simulink model "sampleModel153_pp"  (R2021a)
settings: Solver=VariableStepAuto  StartTime=0.0  StopTime=10.0  RelTol=1e-3
undefined symbols (not defined in the file or in its folder): DiscIntNeverNeededParam, magnitude, Newton, Raphson
libraries: simulink x48, pid_lib x19
(part 2 of 3)

== system sampleModel153_pp/cfblk50/cfblk11 ==
  cfblk1 : Inport
  cfblk12 : Inport  Port=2
  cfblk13 : Inport  Port=3
  cfblk10 : Polyval  Coefs=[ +2.081618890e-019, -1.441693666e-014, +4.719686976e-010, -8.536869453e-006, +1.621573104e-001, -8.087801117e+001 ]
  cfblk11 : Constant  Value=[984784884.031660]  SampleTime=1
  cfblk16 : Delay  SampleTime=1
  cfblk3 : DiscreteFir  SampleTime=1
  cfblk4 : pid_lib/PID Controller  Controller=PID  Form=Parallel  TimeDomain=Discrete-time  UseExternalTs=off  SampleTime=1  IntegratorMethod=Forward Euler  FilterMethod=Forward Euler  ControllerParametersSource=internal  P=1  I=1  D=0  UseFilter=on  N=100  TunerSelectOption=Transfer Function Based (PID Tuner App)  InitialConditionSource=internal  InitialConditionForIntegrator=0  InitialConditionForFilter=0  DifferentiatorICPrevScaledInput=0  ExternalReset=none  TrackingMode=off  Kt=1  LimitOutput=off  SatLimitsSource=internal  UpperSaturationLimit=inf  LowerSaturationLimit=-inf  LinearizeAsGain=off  AntiWindupMode=none  Kb=1  POutMin=[]  POutMax=[]  IOutMin=[]  IOutMax=[]  DOutMin=[]  DOutMax=[]  NOutMin=[]  NOutMax=[]  SumOutMin=[]  SumOutMax=[]  SaturationOutMin=[]  SaturationOutMax=[]  PParamMin=[]  PParamMax=[]  IParamMin=[]  IParamMax=[]  DParamMin=[]  DParamMax=[]  NParamMin=[]  NParamMax=[]  KbParamMin=[]  KbParamMax=[]  KtParamMin=[]  KtParamMax=[]  KbOutMin=[]  KbOutMax=[]  KtOutMin=[]  KtOutMax=[]  IntegratorOutMin=[]  IntegratorOutMax=[]  FilterOutMin=[]  FilterOutMax=[]  SumI1OutMin=[]  SumI1OutMax=[]  SumI2OutMin=[]  SumI2OutMax=[]  SumI3OutMin=[]  SumI3OutMax=[]  SumI4OutMin=[]  SumI4OutMax=[]  SumDOutMin=[]  SumDOutMax=[]  DifferentiatorOutMin=[]  DifferentiatorOutMax=[]  FilterDiffOutCoefMin=[]  FilterDiffOutCoefMax=[]  ReciprocalOutMin=[]  ReciprocalOutMax=[]  SumDenOutMin=[]  SumDenOutMax=[]  SumNumOutMin=[]  SumNumOutMax=[]  DivideOutMin=[]  DivideOutMax=[]  UdiffTsProdOutMin=[]  UdiffTsProdOutMax=[]  NTsProdOutMin=[]  NTsProdOutMax=[]  UintegralTsProdOutMin=[]  UintegralTsProdOutMax=[]  UngainTsProdOutMin=[]  UngainTsProdOutMax=[]  IntegratorContinuousStateAttributes=''  IntegratorStateMustResolveToSignalObject=off  IntegratorRTWStateStorageClass=Auto  FilterContinuousStateAttributes=''  FilterStateMustResolveToSignalObject=off  FilterRTWStateStorageClass=Auto  ParallelPVariant=InternalParameters  IdealPVariant=Disabled  IVariant=InternalParameters  DVariant=InternalParameters  IntegratorVariant=Discrete  SatVariant=Disabled  AWVariant=Passthrough  PCopyVariant=Disabled  TRVariant=Disabled  FdbkBlocksVariant=Forward  IdealPFdbkVariant=Disabled  SatFdbkVariant=Disabled  DerivativeFilterVariant=ForwardEulerFilter  NVariant=InternalParameters  NCopyVariant=Disabled  FilterICVariant=InternalICsFilter  IntegratorICVariant=InternalICs  ExternalResetVariant=Disabled  TRSumVariant=Passthrough  SumFdbkVariant=Disabled  SumVariant=Sum_PID  TsampFilterVariant=InternalTs  TsampNgainVariant=Passthrough  TsampIntegralVariant=Passthrough  ExternalSaturationOutDataTypeStr=Inherit: Same as second input
  cfblk5 : Sqrt  Operator=rSqrt  AlgorithmType=Newton-Raphson  SaturateOnIntegerOverflow=on
  cfblk6 : Rounding
  cfblk7 : Trigonometry
  cfblk8 : Assignment  DiagnosticForDimensions=Warning  IndexOptions=Index vector (dialog)  Indices=1  OutputSizes=1
  cfblk9 : MinMax  Function=max  Inputs=3
  cfblk2 : Outport
  cfblk14 : Outport  Port=2
  cfblk15 : Outport  Port=3
  wires:
  cfblk9/1 -> cfblk7/1
  cfblk13/1 -> cfblk2/1, cfblk10/1
  cfblk3/1 -> cfblk6/1
  cfblk6/1 -> cfblk4/1
  cfblk7/1 -> cfblk3/1
  cfblk12/1 -> cfblk8/1
  cfblk8/1 -> cfblk14/1
  cfblk5/1 -> cfblk8/2, cfblk9/3
  cfblk11/1 -> cfblk5/1
  cfblk1/1 -> cfblk9/1
  cfblk10/1 -> cfblk15/1
  cfblk4/1 -> cfblk16/1
  cfblk16/1 -> cfblk9/2

== system sampleModel153_pp/cfblk50/cfblk12 ==
  cfblk1 : Inport
  cfblk6 : Inport  Port=2
  cfblk3 : ComplexToMagnitudeAngle
  cfblk4 : Sqrt  SaturateOnIntegerOverflow=on
  cfblk5 : Constant  Value=[784222479.091064]  SampleTime=1
  cfblk2 : Outport
  cfblk7 : Outport  Port=2
  wires:
  cfblk1/1 -> cfblk4/1
  cfblk6/1 -> cfblk3/1
  cfblk3/1 -> cfblk7/1
  cfblk3/2 -> cfblk2/1

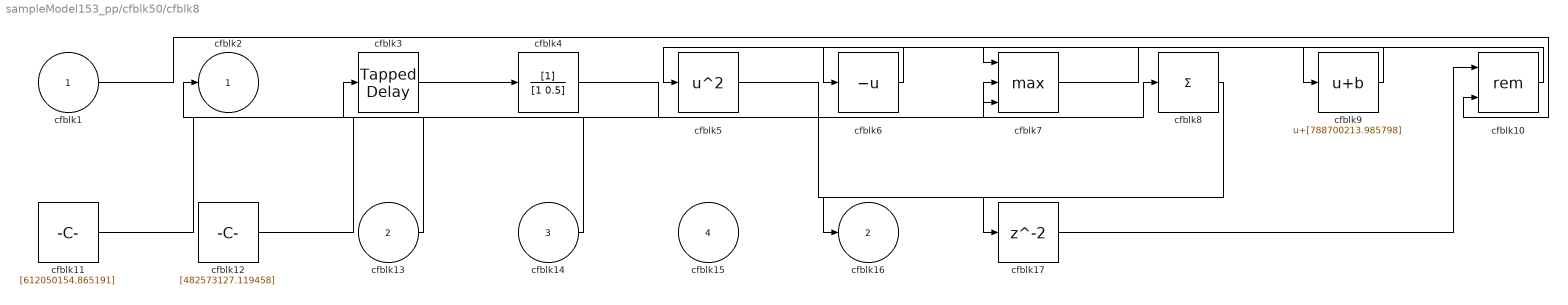
== system sampleModel153_pp/cfblk50/cfblk8 ==
  cfblk1 : Inport
  cfblk13 : Inport  Port=2
  cfblk14 : Inport  Port=3
  cfblk15 : Inport  Port=4
  cfblk10 : Math  Operator=rem  SaturateOnIntegerOverflow=on
  cfblk11 : Constant  Value=[612050154.865191]  SampleTime=1
  cfblk12 : Constant  Value=[482573127.119458]  SampleTime=1
  cfblk17 : Delay  SampleTime=1
  cfblk3 : simulink/Discrete/Tapped Delay  vinit=0.0  samptime=-1  NumDelays=1  DelayOrder=Oldest  includeCurrent=off
  cfblk4 : DiscreteFilter  SampleTime=1
  cfblk5 : Math  Operator=square  SaturateOnIntegerOverflow=on
  cfblk6 : UnaryMinus
  cfblk7 : MinMax  Function=max  Inputs=3
  cfblk8 : Sum  Inputs=+
  cfblk9 : Bias  Bias=[788700213.985798]
  cfblk2 : Outport
  cfblk16 : Outport  Port=2
  wires:
  cfblk11/1 -> cfblk8/1
  cfblk6/1 -> cfblk5/1
  cfblk3/1 -> cfblk4/1
  cfblk10/1 -> cfblk7/1
  cfblk12/1 -> cfblk7/2
  cfblk8/1 -> cfblk16/1
  cfblk14/1 -> cfblk3/1
  cfblk4/1 -> cfblk7/3
  cfblk7/1 -> cfblk9/1
  cfblk9/1 -> cfblk6/1
  cfblk13/1 -> cfblk2/1
  cfblk1/1 -> cfblk10/2
  cfblk5/1 -> cfblk17/1
  cfblk17/1 -> cfblk10/1

== system sampleModel153_pp/cfblk50/cfblk9 ==
  cfblk1 : Inport
  cfblk3 : DiscreteIntegrator  ICPrevOutput=DiscIntNeverNeededParam  ICPrevScaledInput=DiscIntNeverNeededParam
  cfblk4 : Delay  ShowEnablePort=on  SampleTime=1
      settings: InputPortMap=u0,e6
  cfblk5 : DiscreteFir  SampleTime=1
  cfblk6 : DiscreteIntegrator  ICPrevOutput=DiscIntNeverNeededParam  ICPrevScaledInput=DiscIntNeverNeededParam
  cfblk7 : PermuteDimensions
  cfblk8 : Delay  SampleTime=1
  cfblk2 : Outport
  wires:
  cfblk5/1 -> cfblk2/1
  cfblk4/1 -> cfblk3/1
  cfblk7/1 -> cfblk4/1
  cfblk1/1 -> cfblk7/1
  cfblk6/1 -> cfblk5/1, cfblk8/1
  cfblk3/1 -> cfblk6/1
  cfblk8/1 -> cfblk4/2

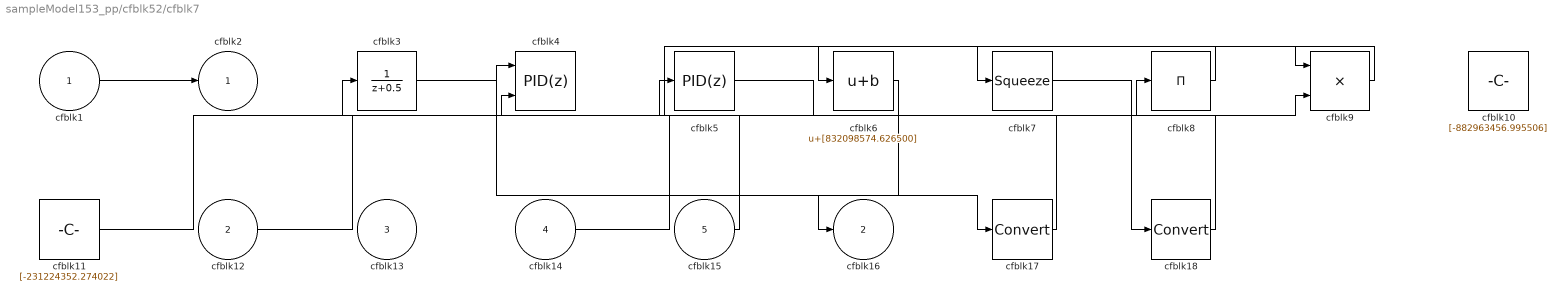
== system sampleModel153_pp/cfblk52/cfblk7 ==
  cfblk1 : Inport
  cfblk12 : Inport  Port=2
  cfblk13 : Inport  Port=3
  cfblk14 : Inport  Port=4
  cfblk15 : Inport  Port=5
  cfblk10 : Constant  Value=[-882963456.995506]  SampleTime=1
  cfblk11 : Constant  Value=[-231224352.274022]  SampleTime=1
  cfblk17 : DataTypeConversion
  cfblk18 : DataTypeConversion
  cfblk3 : DiscreteTransferFcn  SampleTime=1
  cfblk4 : pid_lib/PID Controller (2DOF)  Controller=PID  Form=Parallel  TimeDomain=Discrete-time  UseExternalTs=off  SampleTime=1  IntegratorMethod=Forward Euler  FilterMethod=Forward Euler  ControllerParametersSource=internal  P=1  I=1  D=0  UseFilter=on  N=100  b=1  c=1  TunerSelectOption=Transfer Function Based (PID Tuner App)  InitialConditionSource=internal  InitialConditionForIntegrator=0  InitialConditionForFilter=0  DifferentiatorICPrevScaledInput=0  ExternalReset=none  TrackingMode=off  Kt=1  LimitOutput=off  SatLimitsSource=internal  UpperSaturationLimit=inf  LowerSaturationLimit=-inf  LinearizeAsGain=off  AntiWindupMode=none  Kb=1  POutMin=[]  POutMax=[]  IOutMin=[]  IOutMax=[]  DOutMin=[]  DOutMax=[]  NOutMin=[]  NOutMax=[]  bOutMin=[]  bOutMax=[]  cOutMin=[]  cOutMax=[]  SumOutMin=[]  SumOutMax=[]  SaturationOutMin=[]  SaturationOutMax=[]  PParamMin=[]  PParamMax=[]  IParamMin=[]  IParamMax=[]  DParamMin=[]  DParamMax=[]  NParamMin=[]  NParamMax=[]  bParamMin=[]  bParamMax=[]  cParamMin=[]  cParamMax=[]  KbParamMin=[]  KbParamMax=[]  KtParamMin=[]  KtParamMax=[]  KbOutMin=[]  KbOutMax=[]  KtOutMin=[]  KtOutMax=[]  IntegratorOutMin=[]  IntegratorOutMax=[]  FilterOutMin=[]  FilterOutMax=[]  SumI1OutMin=[]  SumI1OutMax=[]  SumI2OutMin=[]  SumI2OutMax=[]  SumI3OutMin=[]  SumI3OutMax=[]  SumI4OutMin=[]  SumI4OutMax=[]  SumDOutMin=[]  SumDOutMax=[]  Sum1OutMin=[]  Sum1OutMax=[]  Sum2OutMin=[]  Sum2OutMax=[]  Sum3OutMin=[]  Sum3OutMax=[]  DifferentiatorOutMin=[]  DifferentiatorOutMax=[]  FilterDiffOutCoefMin=[]  FilterDiffOutCoefMax=[]  ReciprocalOutMin=[]  ReciprocalOutMax=[]  SumDenOutMin=[]  SumDenOutMax=[]  SumNumOutMin=[]  SumNumOutMax=[]  DivideOutMin=[]  DivideOutMax=[]  UdiffTsProdOutMin=[]  UdiffTsProdOutMax=[]  NTsProdOutMin=[]  NTsProdOutMax=[]  UintegralTsProdOutMin=[]  UintegralTsProdOutMax=[]  UngainTsProdOutMin=[]  UngainTsProdOutMax=[]  IntegratorContinuousStateAttributes=''  IntegratorStateMustResolveToSignalObject=off  IntegratorRTWStateStorageClass=Auto  FilterContinuousStateAttributes=''  FilterStateMustResolveToSignalObject=off  FilterRTWStateStorageClass=Auto  ParallelPVariant=InternalParameters  IdealPVariant=Disabled  IVariant=InternalParameters  DVariant=InternalParameters  bVariant=InternalParameters  cVariant=InternalParameters  IntegratorVariant=Discrete  SatVariant=Disabled  AWVariant=Passthrough  PCopyVariant=Disabled  TRVariant=Disabled  FdbkBlocksVariant=Forward  IdealPFdbkVariant=Disabled  SatFdbkVariant=Disabled  DerivativeFilterVariant=ForwardEulerFilter  NVariant=InternalParameters  NCopyVariant=Disabled  FilterICVariant=InternalICsFilter  IntegratorICVariant=InternalICs  ExternalResetVariant=Disabled  TRSumVariant=Passthrough  SumFdbkVariant=Disabled  SumVariant=Sum_PID  TsampFilterVariant=InternalTs  TsampNgainVariant=Passthrough  TsampIntegralVariant=Passthrough  ExternalSaturationOutDataTypeStr=Inherit: Same as second input
      settings: SourceProductBaseCode=SL
  cfblk5 : pid_lib/PID Controller  Controller=PID  Form=Parallel  TimeDomain=Discrete-time  UseExternalTs=off  SampleTime=1  IntegratorMethod=Forward Euler  FilterMethod=Forward Euler  ControllerParametersSource=internal  P=1  I=1  D=0  UseFilter=on  N=100  TunerSelectOption=Transfer Function Based (PID Tuner App)  InitialConditionSource=internal  InitialConditionForIntegrator=0  InitialConditionForFilter=0  DifferentiatorICPrevScaledInput=0  ExternalReset=none  TrackingMode=off  Kt=1  LimitOutput=off  SatLimitsSource=internal  UpperSaturationLimit=inf  LowerSaturationLimit=-inf  LinearizeAsGain=off  AntiWindupMode=none  Kb=1  POutMin=[]  POutMax=[]  IOutMin=[]  IOutMax=[]  DOutMin=[]  DOutMax=[]  NOutMin=[]  NOutMax=[]  SumOutMin=[]  SumOutMax=[]  SaturationOutMin=[]  SaturationOutMax=[]  PParamMin=[]  PParamMax=[]  IParamMin=[]  IParamMax=[]  DParamMin=[]  DParamMax=[]  NParamMin=[]  NParamMax=[]  KbParamMin=[]  KbParamMax=[]  KtParamMin=[]  KtParamMax=[]  KbOutMin=[]  KbOutMax=[]  KtOutMin=[]  KtOutMax=[]  IntegratorOutMin=[]  IntegratorOutMax=[]  FilterOutMin=[]  FilterOutMax=[]  SumI1OutMin=[]  SumI1OutMax=[]  SumI2OutMin=[]  SumI2OutMax=[]  SumI3OutMin=[]  SumI3OutMax=[]  SumI4OutMin=[]  SumI4OutMax=[]  SumDOutMin=[]  SumDOutMax=[]  DifferentiatorOutMin=[]  DifferentiatorOutMax=[]  FilterDiffOutCoefMin=[]  FilterDiffOutCoefMax=[]  ReciprocalOutMin=[]  ReciprocalOutMax=[]  SumDenOutMin=[]  SumDenOutMax=[]  SumNumOutMin=[]  SumNumOutMax=[]  DivideOutMin=[]  DivideOutMax=[]  UdiffTsProdOutMin=[]  UdiffTsProdOutMax=[]  NTsProdOutMin=[]  NTsProdOutMax=[]  UintegralTsProdOutMin=[]  UintegralTsProdOutMax=[]  UngainTsProdOutMin=[]  UngainTsProdOutMax=[]  IntegratorContinuousStateAttributes=''  IntegratorStateMustResolveToSignalObject=off  IntegratorRTWStateStorageClass=Auto  FilterContinuousStateAttributes=''  FilterStateMustResolveToSignalObject=off  FilterRTWStateStorageClass=Auto  ParallelPVariant=InternalParameters  IdealPVariant=Disabled  IVariant=InternalParameters  DVariant=InternalParameters  IntegratorVariant=Discrete  SatVariant=Disabled  AWVariant=Passthrough  PCopyVariant=Disabled  TRVariant=Disabled  FdbkBlocksVariant=Forward  IdealPFdbkVariant=Disabled  SatFdbkVariant=Disabled  DerivativeFilterVariant=ForwardEulerFilter  NVariant=InternalParameters  NCopyVariant=Disabled  FilterICVariant=InternalICsFilter  IntegratorICVariant=InternalICs  ExternalResetVariant=Disabled  TRSumVariant=Passthrough  SumFdbkVariant=Disabled  SumVariant=Sum_PID  TsampFilterVariant=InternalTs  TsampNgainVariant=Passthrough  TsampIntegralVariant=Passthrough  ExternalSaturationOutDataTypeStr=Inherit: Same as second input
  cfblk6 : Bias  Bias=[832098574.626500]
  cfblk7 : Squeeze
  cfblk8 : Product  Inputs=*
  cfblk9 : Product  Inputs=**
  cfblk2 : Outport
  cfblk16 : Outport  Port=2
  wires:
  cfblk14/1 -> cfblk8/1
  cfblk12/1 -> cfblk9/1
  cfblk6/1 -> cfblk16/1
  cfblk15/1 -> cfblk5/1
  cfblk1/1 -> cfblk2/1
  cfblk9/1 -> cfblk6/1
  cfblk11/1 -> cfblk4/2
  cfblk8/1 -> cfblk7/1
  cfblk5/1 -> cfblk9/2
  cfblk3/1 -> cfblk17/1
  cfblk17/1 -> cfblk4/1
  cfblk7/1 -> cfblk18/1
  cfblk18/1 -> cfblk3/1

== system sampleModel153_pp/cfblk53/cfblk11 ==
  cfblk1 : Inport
  cfblk9 : Inport  Port=2
  cfblk10 : Inport  Port=3
  cfblk11 : Inport  Port=4
  cfblk3 : DiscreteZeroPole  Poles=[0 0.5]  Gain=1
  cfblk4 : pid_lib/PID Controller  Controller=PID  Form=Parallel  TimeDomain=Discrete-time  UseExternalTs=off  SampleTime=1  IntegratorMethod=Forward Euler  FilterMethod=Forward Euler  ControllerParametersSource=internal  P=1  I=1  D=0  UseFilter=on  N=100  TunerSelectOption=Transfer Function Based (PID Tuner App)  InitialConditionSource=internal  InitialConditionForIntegrator=0  InitialConditionForFilter=0  DifferentiatorICPrevScaledInput=0  ExternalReset=none  TrackingMode=off  Kt=1  LimitOutput=off  SatLimitsSource=internal  UpperSaturationLimit=inf  LowerSaturationLimit=-inf  LinearizeAsGain=off  AntiWindupMode=none  Kb=1  POutMin=[]  POutMax=[]  IOutMin=[]  IOutMax=[]  DOutMin=[]  DOutMax=[]  NOutMin=[]  NOutMax=[]  SumOutMin=[]  SumOutMax=[]  SaturationOutMin=[]  SaturationOutMax=[]  PParamMin=[]  PParamMax=[]  IParamMin=[]  IParamMax=[]  DParamMin=[]  DParamMax=[]  NParamMin=[]  NParamMax=[]  KbParamMin=[]  KbParamMax=[]  KtParamMin=[]  KtParamMax=[]  KbOutMin=[]  KbOutMax=[]  KtOutMin=[]  KtOutMax=[]  IntegratorOutMin=[]  IntegratorOutMax=[]  FilterOutMin=[]  FilterOutMax=[]  SumI1OutMin=[]  SumI1OutMax=[]  SumI2OutMin=[]  SumI2OutMax=[]  SumI3OutMin=[]  SumI3OutMax=[]  SumI4OutMin=[]  SumI4OutMax=[]  SumDOutMin=[]  SumDOutMax=[]  DifferentiatorOutMin=[]  DifferentiatorOutMax=[]  FilterDiffOutCoefMin=[]  FilterDiffOutCoefMax=[]  ReciprocalOutMin=[]  ReciprocalOutMax=[]  SumDenOutMin=[]  SumDenOutMax=[]  SumNumOutMin=[]  SumNumOutMax=[]  DivideOutMin=[]  DivideOutMax=[]  UdiffTsProdOutMin=[]  UdiffTsProdOutMax=[]  NTsProdOutMin=[]  NTsProdOutMax=[]  UintegralTsProdOutMin=[]  UintegralTsProdOutMax=[]  UngainTsProdOutMin=[]  UngainTsProdOutMax=[]  IntegratorContinuousStateAttributes=''  IntegratorStateMustResolveToSignalObject=off  IntegratorRTWStateStorageClass=Auto  FilterContinuousStateAttributes=''  FilterStateMustResolveToSignalObject=off  FilterRTWStateStorageClass=Auto  ParallelPVariant=InternalParameters  IdealPVariant=Disabled  IVariant=InternalParameters  DVariant=InternalParameters  IntegratorVariant=Discrete  SatVariant=Disabled  AWVariant=Passthrough  PCopyVariant=Disabled  TRVariant=Disabled  FdbkBlocksVariant=Forward  IdealPFdbkVariant=Disabled  SatFdbkVariant=Disabled  DerivativeFilterVariant=ForwardEulerFilter  NVariant=InternalParameters  NCopyVariant=Disabled  FilterICVariant=InternalICsFilter  IntegratorICVariant=InternalICs  ExternalResetVariant=Disabled  TRSumVariant=Passthrough  SumFdbkVariant=Disabled  SumVariant=Sum_PID  TsampFilterVariant=InternalTs  TsampNgainVariant=Passthrough  TsampIntegralVariant=Passthrough  ExternalSaturationOutDataTypeStr=Inherit: Same as second input
  cfblk5 : Abs
  cfblk6 : Sum  Inputs=|++
  cfblk7 : Signum
  cfblk8 : Abs
  cfblk2 : Outport
  cfblk12 : Outport  Port=2
  wires:
  cfblk9/1 -> cfblk8/1
  cfblk5/1 -> cfblk12/1
  cfblk8/1 -> cfblk4/1
  cfblk1/1 -> cfblk3/1
  cfblk3/1 -> cfblk6/1
  cfblk11/1 -> cfblk7/1
  cfblk4/1 -> cfblk2/1
  cfblk6/1 -> cfblk5/1
  cfblk10/1 -> cfblk6/2

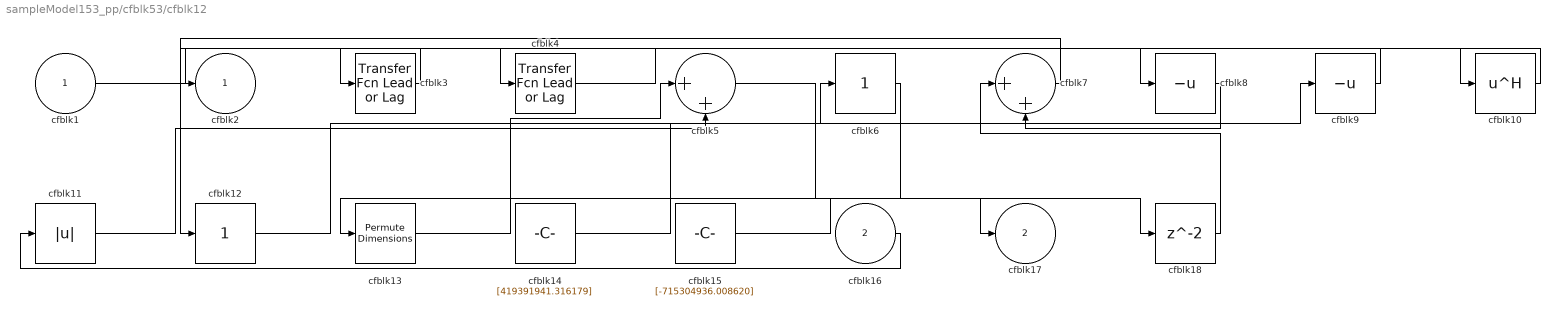
== system sampleModel153_pp/cfblk53/cfblk12 ==
  cfblk1 : Inport
  cfblk16 : Inport  Port=2
  cfblk10 : Math  Operator=hermitian  SaturateOnIntegerOverflow=on
  cfblk11 : Abs
  cfblk12 : simulink/Math Operations/Slider Gain  gain=1  low=0  high=2
  cfblk13 : PermuteDimensions
  cfblk14 : Constant  Value=[419391941.316179]  SampleTime=1
  cfblk15 : Constant  Value=[-715304936.008620]  SampleTime=1
  cfblk18 : Delay  SampleTime=1
  cfblk3 : simulink/Discrete/Transfer Fcn Lead or Lag  PoleZ=0.95  ZeroZ=0.75  ICPrevOutput=0.0  ICPrevInput=0.0  DoSatur=off
      settings: SourceProductBaseCode=SL
  cfblk4 : simulink/Discrete/Transfer Fcn Lead or Lag  PoleZ=0.95  ZeroZ=0.75  ICPrevOutput=0.0  ICPrevInput=0.0  DoSatur=off
      settings: SourceProductBaseCode=SL
  cfblk5 : Sum  Inputs=|++
  cfblk6 : simulink/Math Operations/Slider Gain  gain=1  low=0  high=2
  cfblk7 : Sum  Inputs=|++
  cfblk8 : UnaryMinus
  cfblk9 : UnaryMinus
  cfblk2 : Outport
  cfblk17 : Outport  Port=2
  wires:
  cfblk6/1 -> cfblk13/1
  cfblk16/1 -> cfblk11/1
  cfblk7/1 -> cfblk12/1
  cfblk1/1 -> cfblk4/1
  cfblk12/1 -> cfblk6/1
  cfblk14/1 -> cfblk9/1
  cfblk13/1 -> cfblk5/1
  cfblk11/1 -> cfblk5/2
  cfblk10/1 -> cfblk8/1
  cfblk9/1 -> cfblk3/1
  cfblk3/1 -> cfblk2/1
  cfblk8/1 -> cfblk7/2
  cfblk4/1 -> cfblk10/1
  cfblk15/1 -> cfblk17/1
  cfblk5/1 -> cfblk18/1
  cfblk18/1 -> cfblk7/1

== system sampleModel153_pp/cfblk53/cfblk13 ==
  cfblk1 : Inport
  cfblk12 : Inport  Port=2
  cfblk10 : Sum  Inputs=|++
  cfblk11 : Sum  Inputs=-+
  cfblk14 : Delay  SampleTime=1
  cfblk15 : Delay  SampleTime=1
  cfblk3 : DiscreteFilter  SampleTime=1
  cfblk4 : Delay  DelayLengthSource=Input port  SampleTime=1
      settings: InputPortMap=u0,p1
  cfblk5 : simulink/Math Operations/Slider Gain  gain=1  low=0  high=2
  cfblk6 : Signum
  cfblk7 : simulink/Math Operations/Slider Gain  gain=1  low=0  high=2
  cfblk8 : MinMax  Function=max
  cfblk9 : Gain  Gain=[-990877030.990551]
  cfblk2 : Outport
  cfblk13 : Outport  Port=2
  wires:
  cfblk12/1 -> cfblk13/1
  cfblk3/1 -> cfblk7/1
  cfblk4/1 -> cfblk11/1
  cfblk5/1 -> cfblk4/1
  cfblk9/1 -> cfblk3/1, cfblk8/1
  cfblk1/1 -> cfblk5/1, cfblk11/2
  cfblk11/1 -> cfblk10/1
  cfblk6/1 -> cfblk2/1, cfblk14/1
  cfblk10/1 -> cfblk9/1
  cfblk7/1 -> cfblk6/1
  cfblk14/1 -> cfblk10/2
  cfblk8/1 -> cfblk15/1
  cfblk15/1 -> cfblk4/2

== system sampleModel153_pp/cfblk53/cfblk14 ==
  cfblk1 : Inport
  cfblk6 : Inport  Port=2
  cfblk7 : Inport  Port=3
  cfblk3 : Rounding
  cfblk4 : PermuteDimensions
  cfblk5 : Abs
  cfblk2 : Outport
  cfblk8 : Outport  Port=2
  cfblk9 : Outport  Port=3
  cfblk10 : Outport  Port=4
  wires:
  cfblk1/1 -> cfblk5/1
  cfblk6/1 -> cfblk3/1, cfblk8/1
  cfblk4/1 -> cfblk2/1
  cfblk7/1 -> cfblk4/1
  cfblk5/1 -> cfblk9/1
  cfblk3/1 -> cfblk10/1

== system sampleModel153_pp/cfblk54/cfblk10 ==
  cfblk1 : Inport
  cfblk6 : Inport  Port=2
  cfblk7 : Inport  Port=3
  cfblk3 : simulink/Math Operations/MinMax Running Resettable  Function=min  vinit=0.0
  cfblk4 : Math  Operator=10^u  SaturateOnIntegerOverflow=on
  cfblk5 : Constant  Value=[175787180.328287]  SampleTime=1
  cfblk2 : Outport
  wires:
  cfblk5/1 -> cfblk4/1
  cfblk1/1 -> cfblk2/1
  cfblk4/1 -> cfblk3/1
  cfblk7/1 -> cfblk3/2

== system sampleModel153_pp/cfblk54/cfblk9 ==
  cfblk1 : Inport
  cfblk7 : Inport  Port=2
  cfblk8 : Inport  Port=3
  cfblk9 : Inport  Port=4
  cfblk3 : MinMax
  cfblk4 : Sum  Inputs=+-
  cfblk5 : Constant  Value=[696083638.392896]  SampleTime=1
  cfblk6 : Constant  Value=[-943413520.020544]  SampleTime=1
  cfblk2 : Outport
  wires:
  cfblk4/1 -> cfblk3/1
  cfblk3/1 -> cfblk2/1
  cfblk1/1 -> cfblk4/1
  cfblk5/1 -> cfblk4/2

== system sampleModel153_pp/cfblk55/cfblk10 ==
  cfblk1 : Inport
  cfblk8 : Inport  Port=2
  cfblk3 : Sum  Inputs=+-
  cfblk4 : Sum  Inputs=+
  cfblk5 : MinMax  Function=max
  cfblk6 : Constant  Value=[519421794.730355]  SampleTime=1
  cfblk7 : Constant  Value=[668195430.515494]  SampleTime=1
  cfblk2 : Outport
  wires:
  cfblk7/1 -> cfblk2/1
  cfblk4/1 -> cfblk5/1
  cfblk6/1 -> cfblk4/1
  cfblk8/1 -> cfblk3/1
  cfblk1/1 -> cfblk3/2

== system sampleModel153_pp/cfblk55/cfblk7 ==
  cfblk1 : Inport
  cfblk9 : Inport  Port=2
  cfblk10 : Inport  Port=3
  cfblk11 : Inport  Port=4
  cfblk12 : Inport  Port=5
  cfblk3 : simulink/Discrete/Difference  ICPrevInput=0.0  OutMin=[]  OutMax=[]  OutDataTypeStr=Inherit: Inherit via back propagation  OutDataType=fixdt(1, 16)  OutScaling=2^-10  DoSatur=off
  cfblk4 : Sum  Inputs=+
  cfblk5 : Sum  Inputs=--
  cfblk6 : ComplexToMagnitudeAngle
  cfblk7 : Rounding
  cfblk8 : Reshape
  cfblk2 : Outport
  cfblk13 : Outport  Port=2
  wires:
  cfblk9/1 -> cfblk7/1
  cfblk4/1 -> cfblk6/1
  cfblk8/1 -> cfblk5/1
  cfblk12/1 -> cfblk4/1
  cfblk11/1 -> cfblk3/1
  cfblk1/1 -> cfblk13/1
  cfblk3/1 -> cfblk5/2
  cfblk6/1 -> cfblk8/1
  cfblk10/1 -> cfblk2/1

== system sampleModel153_pp/cfblk55/cfblk8 ==
  cfblk1 : Inport
  cfblk9 : Inport  Port=2
  cfblk12 : Delay  SampleTime=1
  cfblk3 : Rounding
  cfblk4 : Gain  Gain=[218095897.215768]
  cfblk5 : Rounding
  cfblk6 : ComplexToMagnitudeAngle
  cfblk7 : Product  Inputs=*
  cfblk8 : Sum  Inputs=|++
  cfblk2 : Outport
  cfblk10 : Outport  Port=2
  cfblk11 : Outport  Port=3
  wires:
  cfblk8/1 -> cfblk7/1
  cfblk1/1 -> cfblk4/1
  cfblk6/1 -> cfblk3/1
  cfblk6/2 -> cfblk10/1
  cfblk3/1 -> cfblk8/1
  cfblk7/1 -> cfblk5/1, cfblk2/1
  cfblk4/1 -> cfblk6/1
  cfblk9/1 -> cfblk11/1
  cfblk5/1 -> cfblk12/1
  cfblk12/1 -> cfblk8/2

== system sampleModel153_pp/cfblk55/cfblk9 ==
  cfblk1 : Inport
  cfblk9 : Inport  Port=2
  cfblk10 : Inport  Port=3
  cfblk11 : Inport  Port=4
  cfblk12 : Inport  Port=5
  cfblk13 : Inport  Port=6
  cfblk3 : pid_lib/PID Controller  Controller=PID  Form=Parallel  TimeDomain=Discrete-time  UseExternalTs=off  SampleTime=1  IntegratorMethod=Forward Euler  FilterMethod=Forward Euler  ControllerParametersSource=internal  P=1  I=1  D=0  UseFilter=on  N=100  TunerSelectOption=Transfer Function Based (PID Tuner App)  InitialConditionSource=internal  InitialConditionForIntegrator=0  InitialConditionForFilter=0  DifferentiatorICPrevScaledInput=0  ExternalReset=none  TrackingMode=off  Kt=1  LimitOutput=off  SatLimitsSource=internal  UpperSaturationLimit=inf  LowerSaturationLimit=-inf  LinearizeAsGain=off  AntiWindupMode=none  Kb=1  POutMin=[]  POutMax=[]  IOutMin=[]  IOutMax=[]  DOutMin=[]  DOutMax=[]  NOutMin=[]  NOutMax=[]  SumOutMin=[]  SumOutMax=[]  SaturationOutMin=[]  SaturationOutMax=[]  PParamMin=[]  PParamMax=[]  IParamMin=[]  IParamMax=[]  DParamMin=[]  DParamMax=[]  NParamMin=[]  NParamMax=[]  KbParamMin=[]  KbParamMax=[]  KtParamMin=[]  KtParamMax=[]  KbOutMin=[]  KbOutMax=[]  KtOutMin=[]  KtOutMax=[]  IntegratorOutMin=[]  IntegratorOutMax=[]  FilterOutMin=[]  FilterOutMax=[]  SumI1OutMin=[]  SumI1OutMax=[]  SumI2OutMin=[]  SumI2OutMax=[]  SumI3OutMin=[]  SumI3OutMax=[]  SumI4OutMin=[]  SumI4OutMax=[]  SumDOutMin=[]  SumDOutMax=[]  DifferentiatorOutMin=[]  DifferentiatorOutMax=[]  FilterDiffOutCoefMin=[]  FilterDiffOutCoefMax=[]  ReciprocalOutMin=[]  ReciprocalOutMax=[]  SumDenOutMin=[]  SumDenOutMax=[]  SumNumOutMin=[]  SumNumOutMax=[]  DivideOutMin=[]  DivideOutMax=[]  UdiffTsProdOutMin=[]  UdiffTsProdOutMax=[]  NTsProdOutMin=[]  NTsProdOutMax=[]  UintegralTsProdOutMin=[]  UintegralTsProdOutMax=[]  UngainTsProdOutMin=[]  UngainTsProdOutMax=[]  IntegratorContinuousStateAttributes=''  IntegratorStateMustResolveToSignalObject=off  IntegratorRTWStateStorageClass=Auto  FilterContinuousStateAttributes=''  FilterStateMustResolveToSignalObject=off  FilterRTWStateStorageClass=Auto  ParallelPVariant=InternalParameters  IdealPVariant=Disabled  IVariant=InternalParameters  DVariant=InternalParameters  IntegratorVariant=Discrete  SatVariant=Disabled  AWVariant=Passthrough  PCopyVariant=Disabled  TRVariant=Disabled  FdbkBlocksVariant=Forward  IdealPFdbkVariant=Disabled  SatFdbkVariant=Disabled  DerivativeFilterVariant=ForwardEulerFilter  NVariant=InternalParameters  NCopyVariant=Disabled  FilterICVariant=InternalICsFilter  IntegratorICVariant=InternalICs  ExternalResetVariant=Disabled  TRSumVariant=Passthrough  SumFdbkVariant=Disabled  SumVariant=Sum_PID  TsampFilterVariant=InternalTs  TsampNgainVariant=Passthrough  TsampIntegralVariant=Passthrough  ExternalSaturationOutDataTypeStr=Inherit: Same as second input
  cfblk4 : Sqrt  SaturateOnIntegerOverflow=on
  cfblk5 : Sin  TimeSource=Use external signal  SampleTime=0
  cfblk6 : Constant  Value=[-874027630.229869]  SampleTime=1
  cfblk7 : Constant  Value=[-999264160.149922]  SampleTime=1
  cfblk8 : Constant  Value=[958342791.090826]  SampleTime=1
  cfblk2 : Outport
  cfblk14 : Outport  Port=2
  wires:
  cfblk7/1 -> cfblk4/1
  cfblk1/1 -> cfblk5/1
  cfblk12/1 -> cfblk2/1
  cfblk3/1 -> cfblk14/1
  cfblk5/1 -> cfblk3/1

== system sampleModel153_pp/cfblk56/cfblk7 ==
  cfblk1 : Inport
  cfblk10 : Inport  Port=2
  cfblk11 : Inport  Port=3
  cfblk12 : Inport  Port=4
  cfblk13 : Inport  Port=5
  cfblk3 : UnitDelay  HasFrameUpgradeWarning=on
  cfblk4 : Delay  ShowEnablePort=on  SampleTime=1
      settings: InputPortMap=u0,e6
  cfblk5 : simulink/Discrete/Transfer Fcn Real Zero  ZeroZ=0.75  ICPrevInput=0.0  DoSatur=off
      settings: SourceProductBaseCode=SL
  cfblk6 : PermuteDimensions
  cfblk7 : Assignment  DiagnosticForDimensions=Warning  IndexOptions=Index vector (dialog)  Indices=1  OutputSizes=1
  cfblk8 : Constant  Value=[-59489138.603640]  SampleTime=1
  cfblk9 : Constant  Value=[610527409.433895]  SampleTime=1
  cfblk2 : Outport
  wires:
  cfblk3/1 -> cfblk4/1
  cfblk9/1 -> cfblk4/2
  cfblk10/1 -> cfblk5/1
  cfblk12/1 -> cfblk2/1
  cfblk11/1 -> cfblk6/1
  cfblk13/1 -> cfblk7/1
  cfblk4/1 -> cfblk7/2
  cfblk6/1 -> cfblk3/1

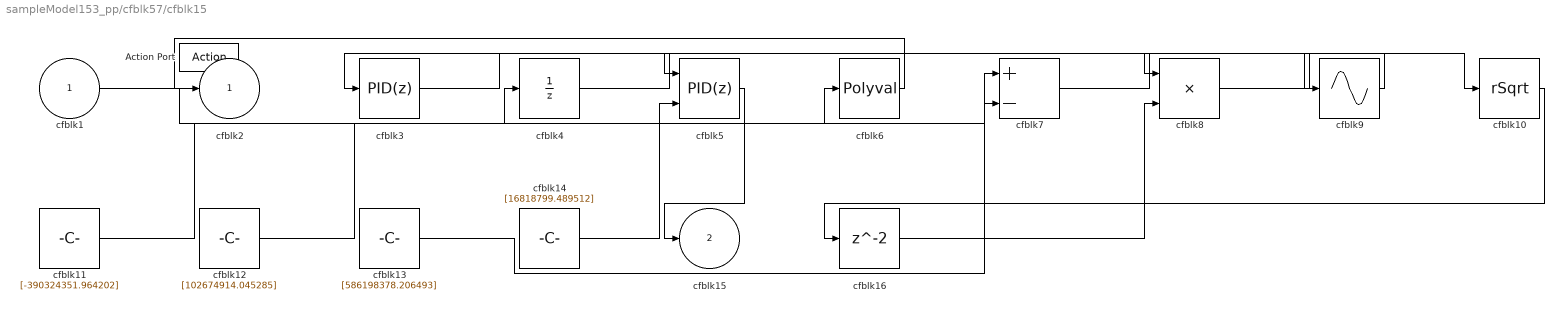
== system sampleModel153_pp/cfblk57/cfblk15 ==
  cfblk1 : Inport
  Action Port : ActionPort  ActionPortLabel=if(u1 >= 0)
  cfblk10 : Sqrt  Operator=rSqrt  AlgorithmType=Newton-Raphson  SaturateOnIntegerOverflow=on
  cfblk11 : Constant  Value=[-390324351.964202]  SampleTime=1
  cfblk12 : Constant  Value=[102674914.045285]  SampleTime=1
  cfblk13 : Constant  Value=[586198378.206493]  SampleTime=1
  cfblk14 : Constant  Value=[16818799.489512]  SampleTime=1
  cfblk16 : Delay
  cfblk3 : pid_lib/PID Controller  Controller=PID  Form=Parallel  TimeDomain=Discrete-time  UseExternalTs=off  SampleTime=-1  IntegratorMethod=Forward Euler  FilterMethod=Forward Euler  ControllerParametersSource=internal  P=1  I=1  D=0  UseFilter=on  N=100  TunerSelectOption=Transfer Function Based (PID Tuner App)  InitialConditionSource=internal  InitialConditionForIntegrator=0  InitialConditionForFilter=0  DifferentiatorICPrevScaledInput=0  ExternalReset=none  TrackingMode=off  Kt=1  LimitOutput=off  SatLimitsSource=internal  UpperSaturationLimit=inf  LowerSaturationLimit=-inf  LinearizeAsGain=off  AntiWindupMode=none  Kb=1  POutMin=[]  POutMax=[]  IOutMin=[]  IOutMax=[]  DOutMin=[]  DOutMax=[]  NOutMin=[]  NOutMax=[]  SumOutMin=[]  SumOutMax=[]  SaturationOutMin=[]  SaturationOutMax=[]  PParamMin=[]  PParamMax=[]  IParamMin=[]  IParamMax=[]  DParamMin=[]  DParamMax=[]  NParamMin=[]  NParamMax=[]  KbParamMin=[]  KbParamMax=[]  KtParamMin=[]  KtParamMax=[]  KbOutMin=[]  KbOutMax=[]  KtOutMin=[]  KtOutMax=[]  IntegratorOutMin=[]  IntegratorOutMax=[]  FilterOutMin=[]  FilterOutMax=[]  SumI1OutMin=[]  SumI1OutMax=[]  SumI2OutMin=[]  SumI2OutMax=[]  SumI3OutMin=[]  SumI3OutMax=[]  SumI4OutMin=[]  SumI4OutMax=[]  SumDOutMin=[]  SumDOutMax=[]  DifferentiatorOutMin=[]  DifferentiatorOutMax=[]  FilterDiffOutCoefMin=[]  FilterDiffOutCoefMax=[]  ReciprocalOutMin=[]  ReciprocalOutMax=[]  SumDenOutMin=[]  SumDenOutMax=[]  SumNumOutMin=[]  SumNumOutMax=[]  DivideOutMin=[]  DivideOutMax=[]  UdiffTsProdOutMin=[]  UdiffTsProdOutMax=[]  NTsProdOutMin=[]  NTsProdOutMax=[]  UintegralTsProdOutMin=[]  UintegralTsProdOutMax=[]  UngainTsProdOutMin=[]  UngainTsProdOutMax=[]  IntegratorContinuousStateAttributes=''  IntegratorStateMustResolveToSignalObject=off  IntegratorRTWStateStorageClass=Auto  FilterContinuousStateAttributes=''  FilterStateMustResolveToSignalObject=off  FilterRTWStateStorageClass=Auto  ParallelPVariant=InternalParameters  IdealPVariant=Disabled  IVariant=InternalParameters  DVariant=InternalParameters  IntegratorVariant=Discrete  SatVariant=Disabled  AWVariant=Passthrough  PCopyVariant=Disabled  TRVariant=Disabled  FdbkBlocksVariant=Forward  IdealPFdbkVariant=Disabled  SatFdbkVariant=Disabled  DerivativeFilterVariant=ForwardEulerFilter  NVariant=InternalParameters  NCopyVariant=Disabled  FilterICVariant=InternalICsFilter  IntegratorICVariant=InternalICs  ExternalResetVariant=Disabled  TRSumVariant=Passthrough  SumFdbkVariant=Disabled  SumVariant=Sum_PID  TsampFilterVariant=InternalTs  TsampNgainVariant=Passthrough  TsampIntegralVariant=Passthrough  ExternalSaturationOutDataTypeStr=Inherit: Same as second input
  cfblk4 : UnitDelay  SampleTime=-1  HasFrameUpgradeWarning=on
  cfblk5 : pid_lib/PID Controller (2DOF)  Controller=PID  Form=Parallel  TimeDomain=Discrete-time  UseExternalTs=off  SampleTime=-1  IntegratorMethod=Forward Euler  FilterMethod=Forward Euler  ControllerParametersSource=internal  P=1  I=1  D=0  UseFilter=on  N=100  b=1  c=1  TunerSelectOption=Transfer Function Based (PID Tuner App)  InitialConditionSource=internal  InitialConditionForIntegrator=0  InitialConditionForFilter=0  DifferentiatorICPrevScaledInput=0  ExternalReset=none  TrackingMode=off  Kt=1  LimitOutput=off  SatLimitsSource=internal  UpperSaturationLimit=inf  LowerSaturationLimit=-inf  LinearizeAsGain=off  AntiWindupMode=none  Kb=1  POutMin=[]  POutMax=[]  IOutMin=[]  IOutMax=[]  DOutMin=[]  DOutMax=[]  NOutMin=[]  NOutMax=[]  bOutMin=[]  bOutMax=[]  cOutMin=[]  cOutMax=[]  SumOutMin=[]  SumOutMax=[]  SaturationOutMin=[]  SaturationOutMax=[]  PParamMin=[]  PParamMax=[]  IParamMin=[]  IParamMax=[]  DParamMin=[]  DParamMax=[]  NParamMin=[]  NParamMax=[]  bParamMin=[]  bParamMax=[]  cParamMin=[]  cParamMax=[]  KbParamMin=[]  KbParamMax=[]  KtParamMin=[]  KtParamMax=[]  KbOutMin=[]  KbOutMax=[]  KtOutMin=[]  KtOutMax=[]  IntegratorOutMin=[]  IntegratorOutMax=[]  FilterOutMin=[]  FilterOutMax=[]  SumI1OutMin=[]  SumI1OutMax=[]  SumI2OutMin=[]  SumI2OutMax=[]  SumI3OutMin=[]  SumI3OutMax=[]  SumI4OutMin=[]  SumI4OutMax=[]  SumDOutMin=[]  SumDOutMax=[]  Sum1OutMin=[]  Sum1OutMax=[]  Sum2OutMin=[]  Sum2OutMax=[]  Sum3OutMin=[]  Sum3OutMax=[]  DifferentiatorOutMin=[]  DifferentiatorOutMax=[]  FilterDiffOutCoefMin=[]  FilterDiffOutCoefMax=[]  ReciprocalOutMin=[]  ReciprocalOutMax=[]  SumDenOutMin=[]  SumDenOutMax=[]  SumNumOutMin=[]  SumNumOutMax=[]  DivideOutMin=[]  DivideOutMax=[]  UdiffTsProdOutMin=[]  UdiffTsProdOutMax=[]  NTsProdOutMin=[]  NTsProdOutMax=[]  UintegralTsProdOutMin=[]  UintegralTsProdOutMax=[]  UngainTsProdOutMin=[]  UngainTsProdOutMax=[]  IntegratorContinuousStateAttributes=''  IntegratorStateMustResolveToSignalObject=off  IntegratorRTWStateStorageClass=Auto  FilterContinuousStateAttributes=''  FilterStateMustResolveToSignalObject=off  FilterRTWStateStorageClass=Auto  ParallelPVariant=InternalParameters  IdealPVariant=Disabled  IVariant=InternalParameters  DVariant=InternalParameters  bVariant=InternalParameters  cVariant=InternalParameters  IntegratorVariant=Discrete  SatVariant=Disabled  AWVariant=Passthrough  PCopyVariant=Disabled  TRVariant=Disabled  FdbkBlocksVariant=Forward  IdealPFdbkVariant=Disabled  SatFdbkVariant=Disabled  DerivativeFilterVariant=ForwardEulerFilter  NVariant=InternalParameters  NCopyVariant=Disabled  FilterICVariant=InternalICsFilter  IntegratorICVariant=InternalICs  ExternalResetVariant=Disabled  TRSumVariant=Passthrough  SumFdbkVariant=Disabled  SumVariant=Sum_PID  TsampFilterVariant=InternalTs  TsampNgainVariant=Passthrough  TsampIntegralVariant=Passthrough  ExternalSaturationOutDataTypeStr=Inherit: Same as second input
      settings: SourceProductBaseCode=SL
  cfblk6 : Polyval  Coefs=[ +2.081618890e-019, -1.441693666e-014, +4.719686976e-010, -8.536869453e-006, +1.621573104e-001, -8.087801117e+001 ]
  cfblk7 : Sum  Inputs=+-
  cfblk8 : Product  Inputs=**
  cfblk9 : Sin  TimeSource=Use external signal  SampleTime=0
  cfblk2 : Outport
  cfblk15 : Outport  Port=2
  wires:
  cfblk11/1 -> cfblk4/1
  cfblk5/1 -> cfblk15/1
  cfblk6/1 -> cfblk2/1
  cfblk8/1 -> cfblk10/1
  cfblk7/1 -> cfblk9/1
  cfblk1/1 -> cfblk6/1
  cfblk9/1 -> cfblk3/1
  cfblk4/1 -> cfblk8/1
  cfblk13/1 -> cfblk7/1
  cfblk12/1 -> cfblk7/2
  cfblk3/1 -> cfblk5/1
  cfblk14/1 -> cfblk5/2
  cfblk10/1 -> cfblk16/1
  cfblk16/1 -> cfblk8/2

== system sampleModel153_pp/cfblk57/cfblk16 ==
  cfblk1 : Inport
  cfblk10 : Inport  Port=2
  cfblk11 : Inport  Port=3
  Action Port : ActionPort  ActionPortLabel=else
  cfblk13 : Delay
  cfblk14 : Delay
  cfblk3 : Delay  ShowEnablePort=on
      settings: InputPortMap=u0,e6
  cfblk4 : simulink/Discrete/Transfer Fcn Lead or Lag  PoleZ=0.95  ZeroZ=0.75  ICPrevOutput=0.0  ICPrevInput=0.0  DoSatur=off
      settings: SourceProductBaseCode=SL
  cfblk5 : Trigonometry
  cfblk6 : Product
  cfblk7 : Sqrt  SaturateOnIntegerOverflow=on
  cfblk8 : Product  Inputs=*
  cfblk9 : MinMax  Inputs=3
  cfblk2 : Outport
  cfblk12 : Outport  Port=2
  wires:
  cfblk5/1 -> cfblk9/1
  cfblk8/1 -> cfblk7/1, cfblk13/1
  cfblk7/1 -> cfblk12/1
  cfblk1/1 -> cfblk2/1
  cfblk3/1 -> cfblk9/3
  cfblk10/1 -> cfblk6/1, cfblk5/1
  cfblk4/1 -> cfblk8/1
  cfblk11/1 -> cfblk6/2
  cfblk9/1 -> cfblk4/1, cfblk14/1
  cfblk6/1 -> cfblk3/1
  cfblk13/1 -> cfblk9/2
  cfblk14/1 -> cfblk3/2

== system sampleModel153_pp/cfblk57/cfblk8 ==
  cfblk1 : Inport
  cfblk11 : Inport  Port=2
  cfblk10 : DotProduct  InputSameDT=on  OutDataTypeStr=Inherit: Inherit via internal rule
  cfblk14 : Delay  SampleTime=1
  cfblk3 : UnitDelay  HasFrameUpgradeWarning=on
  cfblk4 : DiscreteIntegrator  ICPrevOutput=DiscIntNeverNeededParam  ICPrevScaledInput=DiscIntNeverNeededParam
  cfblk5 : DiscreteFir  SampleTime=1
  cfblk6 : UnitDelay  HasFrameUpgradeWarning=on
  cfblk7 : DotProduct  InputSameDT=on  OutDataTypeStr=Inherit: Inherit via internal rule
  cfblk8 : Sqrt  Operator=rSqrt  AlgorithmType=Newton-Raphson  SaturateOnIntegerOverflow=on
  cfblk9 : Polyval  Coefs=[ +2.081618890e-019, -1.441693666e-014, +4.719686976e-010, -8.536869453e-006, +1.621573104e-001, -8.087801117e+001 ]
  cfblk2 : Outport
  cfblk12 : Outport  Port=2
  cfblk13 : Outport  Port=3
  wires:
  cfblk9/1 -> cfblk5/1
  cfblk4/1 -> cfblk3/1
  cfblk11/1 -> cfblk13/1
  cfblk1/1 -> cfblk9/1, cfblk7/2, cfblk10/2
  cfblk8/1 -> cfblk7/1, cfblk14/1
  cfblk5/1 -> cfblk6/1
  cfblk3/1 -> cfblk8/1
  cfblk7/1 -> cfblk2/1
  cfblk10/1 -> cfblk4/1
  cfblk6/1 -> cfblk12/1
  cfblk14/1 -> cfblk10/1

== system sampleModel153_pp/cfblk57/cfblk9 ==
  cfblk1 : Inport
  cfblk9 : Inport  Port=2
  cfblk3 : DiscreteFir  SampleTime=1
  cfblk4 : Math  SaturateOnIntegerOverflow=on
  cfblk5 : Gain  Gain=[514643076.811779]
  cfblk6 : Sqrt  Operator=rSqrt  AlgorithmType=Newton-Raphson  SaturateOnIntegerOverflow=on
  cfblk7 : Constant  Value=[-632687053.672223]  SampleTime=1
  cfblk8 : Constant  Value=[-447542984.857038]  SampleTime=1
  cfblk2 : Outport
  cfblk10 : Outport  Port=2
  cfblk11 : Outport  Port=3
  wires:
  cfblk4/1 -> cfblk10/1
  cfblk6/1 -> cfblk2/1
  cfblk8/1 -> cfblk4/1
  cfblk7/1 -> cfblk6/1
  cfblk5/1 -> cfblk3/1
  cfblk1/1 -> cfblk11/1
  cfblk9/1 -> cfblk5/1

== system sampleModel153_pp/cfblk58/cfblk7 ==
  cfblk1 : Inport
  cfblk10 : Inport  Port=2
  cfblk11 : Inport  Port=3
  cfblk12 : Inport  Port=4
  cfblk13 : Inport  Port=5
  cfblk3 : Squeeze
  cfblk4 : DotProduct  InputSameDT=on  OutDataTypeStr=Inherit: Inherit via internal rule
  cfblk5 : Sum  Inputs=+-
  cfblk6 : Sqrt  Operator=rSqrt  AlgorithmType=Newton-Raphson  SaturateOnIntegerOverflow=on
  cfblk7 : Abs
  cfblk8 : Gain  Gain=[-811579831.073638]
  cfblk9 : Constant  Value=[-423949083.993615]  SampleTime=1
  cfblk2 : Outport
  wires:
  cfblk5/1 -> cfblk8/1
  cfblk10/1 -> cfblk5/1
  cfblk6/1 -> cfblk4/1
  cfblk12/1 -> cfblk3/1
  cfblk11/1 -> cfblk2/1
  cfblk13/1 -> cfblk7/1
  cfblk7/1 -> cfblk5/2
  cfblk3/1 -> cfblk6/1
  cfblk9/1 -> cfblk4/2

== system sampleModel153_pp/cfblk58/cfblk8 ==
  cfblk1 : Inport
  cfblk14 : Inport  Port=2
  cfblk15 : Inport  Port=3
  cfblk10 : Polyval  Coefs=[ +2.081618890e-019, -1.441693666e-014, +4.719686976e-010, -8.536869453e-006, +1.621573104e-001, -8.087801117e+001 ]
  cfblk11 : Signum
  cfblk12 : Constant  Value=[-112483464.536165]  SampleTime=1
  cfblk13 : Constant  Value=[-386105699.936164]  SampleTime=1
  cfblk16 : Delay  SampleTime=1
  cfblk17 : Delay  SampleTime=1
  cfblk3 : pid_lib/PID Controller (2DOF)  Controller=PID  Form=Parallel  TimeDomain=Discrete-time  UseExternalTs=off  SampleTime=1  IntegratorMethod=Forward Euler  FilterMethod=Forward Euler  ControllerParametersSource=internal  P=1  I=1  D=0  UseFilter=on  N=100  b=1  c=1  TunerSelectOption=Transfer Function Based (PID Tuner App)  InitialConditionSource=internal  InitialConditionForIntegrator=0  InitialConditionForFilter=0  DifferentiatorICPrevScaledInput=0  ExternalReset=none  TrackingMode=off  Kt=1  LimitOutput=off  SatLimitsSource=internal  UpperSaturationLimit=inf  LowerSaturationLimit=-inf  LinearizeAsGain=off  AntiWindupMode=none  Kb=1  POutMin=[]  POutMax=[]  IOutMin=[]  IOutMax=[]  DOutMin=[]  DOutMax=[]  NOutMin=[]  NOutMax=[]  bOutMin=[]  bOutMax=[]  cOutMin=[]  cOutMax=[]  SumOutMin=[]  SumOutMax=[]  SaturationOutMin=[]  SaturationOutMax=[]  PParamMin=[]  PParamMax=[]  IParamMin=[]  IParamMax=[]  DParamMin=[]  DParamMax=[]  NParamMin=[]  NParamMax=[]  bParamMin=[]  bParamMax=[]  cParamMin=[]  cParamMax=[]  KbParamMin=[]  KbParamMax=[]  KtParamMin=[]  KtParamMax=[]  KbOutMin=[]  KbOutMax=[]  KtOutMin=[]  KtOutMax=[]  IntegratorOutMin=[]  IntegratorOutMax=[]  FilterOutMin=[]  FilterOutMax=[]  SumI1OutMin=[]  SumI1OutMax=[]  SumI2OutMin=[]  SumI2OutMax=[]  SumI3OutMin=[]  SumI3OutMax=[]  SumI4OutMin=[]  SumI4OutMax=[]  SumDOutMin=[]  SumDOutMax=[]  Sum1OutMin=[]  Sum1OutMax=[]  Sum2OutMin=[]  Sum2OutMax=[]  Sum3OutMin=[]  Sum3OutMax=[]  DifferentiatorOutMin=[]  DifferentiatorOutMax=[]  FilterDiffOutCoefMin=[]  FilterDiffOutCoefMax=[]  ReciprocalOutMin=[]  ReciprocalOutMax=[]  SumDenOutMin=[]  SumDenOutMax=[]  SumNumOutMin=[]  SumNumOutMax=[]  DivideOutMin=[]  DivideOutMax=[]  UdiffTsProdOutMin=[]  UdiffTsProdOutMax=[]  NTsProdOutMin=[]  NTsProdOutMax=[]  UintegralTsProdOutMin=[]  UintegralTsProdOutMax=[]  UngainTsProdOutMin=[]  UngainTsProdOutMax=[]  IntegratorContinuousStateAttributes=''  IntegratorStateMustResolveToSignalObject=off  IntegratorRTWStateStorageClass=Auto  FilterContinuousStateAttributes=''  FilterStateMustResolveToSignalObject=off  FilterRTWStateStorageClass=Auto  ParallelPVariant=InternalParameters  IdealPVariant=Disabled  IVariant=InternalParameters  DVariant=InternalParameters  bVariant=InternalParameters  cVariant=InternalParameters  IntegratorVariant=Discrete  SatVariant=Disabled  AWVariant=Passthrough  PCopyVariant=Disabled  TRVariant=Disabled  FdbkBlocksVariant=Forward  IdealPFdbkVariant=Disabled  SatFdbkVariant=Disabled  DerivativeFilterVariant=ForwardEulerFilter  NVariant=InternalParameters  NCopyVariant=Disabled  FilterICVariant=InternalICsFilter  IntegratorICVariant=InternalICs  ExternalResetVariant=Disabled  TRSumVariant=Passthrough  SumFdbkVariant=Disabled  SumVariant=Sum_PID  TsampFilterVariant=InternalTs  TsampNgainVariant=Passthrough  TsampIntegralVariant=Passthrough  ExternalSaturationOutDataTypeStr=Inherit: Same as second input
      settings: SourceProductBaseCode=SL
  cfblk4 : pid_lib/PID Controller (2DOF)  Controller=PID  Form=Parallel  TimeDomain=Discrete-time  UseExternalTs=off  SampleTime=1  IntegratorMethod=Forward Euler  FilterMethod=Forward Euler  ControllerParametersSource=internal  P=1  I=1  D=0  UseFilter=on  N=100  b=1  c=1  TunerSelectOption=Transfer Function Based (PID Tuner App)  InitialConditionSource=internal  InitialConditionForIntegrator=0  InitialConditionForFilter=0  DifferentiatorICPrevScaledInput=0  ExternalReset=none  TrackingMode=off  Kt=1  LimitOutput=off  SatLimitsSource=internal  UpperSaturationLimit=inf  LowerSaturationLimit=-inf  LinearizeAsGain=off  AntiWindupMode=none  Kb=1  POutMin=[]  POutMax=[]  IOutMin=[]  IOutMax=[]  DOutMin=[]  DOutMax=[]  NOutMin=[]  NOutMax=[]  bOutMin=[]  bOutMax=[]  cOutMin=[]  cOutMax=[]  SumOutMin=[]  SumOutMax=[]  SaturationOutMin=[]  SaturationOutMax=[]  PParamMin=[]  PParamMax=[]  IParamMin=[]  IParamMax=[]  DParamMin=[]  DParamMax=[]  NParamMin=[]  NParamMax=[]  bParamMin=[]  bParamMax=[]  cParamMin=[]  cParamMax=[]  KbParamMin=[]  KbParamMax=[]  KtParamMin=[]  KtParamMax=[]  KbOutMin=[]  KbOutMax=[]  KtOutMin=[]  KtOutMax=[]  IntegratorOutMin=[]  IntegratorOutMax=[]  FilterOutMin=[]  FilterOutMax=[]  SumI1OutMin=[]  SumI1OutMax=[]  SumI2OutMin=[]  SumI2OutMax=[]  SumI3OutMin=[]  SumI3OutMax=[]  SumI4OutMin=[]  SumI4OutMax=[]  SumDOutMin=[]  SumDOutMax=[]  Sum1OutMin=[]  Sum1OutMax=[]  Sum2OutMin=[]  Sum2OutMax=[]  Sum3OutMin=[]  Sum3OutMax=[]  DifferentiatorOutMin=[]  DifferentiatorOutMax=[]  FilterDiffOutCoefMin=[]  FilterDiffOutCoefMax=[]  ReciprocalOutMin=[]  ReciprocalOutMax=[]  SumDenOutMin=[]  SumDenOutMax=[]  SumNumOutMin=[]  SumNumOutMax=[]  DivideOutMin=[]  DivideOutMax=[]  UdiffTsProdOutMin=[]  UdiffTsProdOutMax=[]  NTsProdOutMin=[]  NTsProdOutMax=[]  UintegralTsProdOutMin=[]  UintegralTsProdOutMax=[]  UngainTsProdOutMin=[]  UngainTsProdOutMax=[]  IntegratorContinuousStateAttributes=''  IntegratorStateMustResolveToSignalObject=off  IntegratorRTWStateStorageClass=Auto  FilterContinuousStateAttributes=''  FilterStateMustResolveToSignalObject=off  FilterRTWStateStorageClass=Auto  ParallelPVariant=InternalParameters  IdealPVariant=Disabled  IVariant=InternalParameters  DVariant=InternalParameters  bVariant=InternalParameters  cVariant=InternalParameters  IntegratorVariant=Discrete  SatVariant=Disabled  AWVariant=Passthrough  PCopyVariant=Disabled  TRVariant=Disabled  FdbkBlocksVariant=Forward  IdealPFdbkVariant=Disabled  SatFdbkVariant=Disabled  DerivativeFilterVariant=ForwardEulerFilter  NVariant=InternalParameters  NCopyVariant=Disabled  FilterICVariant=InternalICsFilter  IntegratorICVariant=InternalICs  ExternalResetVariant=Disabled  TRSumVariant=Passthrough  SumFdbkVariant=Disabled  SumVariant=Sum_PID  TsampFilterVariant=InternalTs  TsampNgainVariant=Passthrough  TsampIntegralVariant=Passthrough  ExternalSaturationOutDataTypeStr=Inherit: Same as second input
      settings: SourceProductBaseCode=SL
  cfblk5 : Delay  ShowEnablePort=on  SampleTime=1
      settings: InputPortMap=u0,e6
  cfblk6 : simulink/Discrete/Transfer Fcn Lead or Lag  PoleZ=0.95  ZeroZ=0.75  ICPrevOutput=0.0  ICPrevInput=0.0  DoSatur=off
      settings: SourceProductBaseCode=SL
  cfblk7 : DiscreteFilter  SampleTime=1
  cfblk8 : DiscreteFir  SampleTime=1
  cfblk9 : Delay  ShowEnablePort=on  SampleTime=1
      settings: InputPortMap=u0,e6
  cfblk2 : Outport
  wires:
  cfblk15/1 -> cfblk3/1
  cfblk11/1 -> cfblk5/1
  cfblk13/1 -> cfblk5/2
  cfblk3/1 -> cfblk7/1
  cfblk1/1 -> cfblk2/1
  cfblk12/1 -> cfblk4/1
  cfblk8/1 -> cfblk10/1
  cfblk14/1 -> cfblk6/1
  cfblk10/1 -> cfblk9/1
  cfblk6/1 -> cfblk9/2
  cfblk7/1 -> cfblk8/1
  cfblk4/1 -> cfblk11/1
  cfblk9/1 -> cfblk16/1
  cfblk16/1 -> cfblk3/2
  cfblk5/1 -> cfblk17/1
  cfblk17/1 -> cfblk4/2

== system sampleModel153_pp/cfblk58/cfblk9 ==
  cfblk1 : Inport
  cfblk8 : Inport  Port=2
  cfblk9 : Inport  Port=3
  cfblk10 : Inport  Port=4
  cfblk3 : Assignment  DiagnosticForDimensions=Warning  IndexOptions=Index vector (dialog)  Indices=1  OutputSizes=1
  cfblk4 : Assignment  DiagnosticForDimensions=Warning  IndexOptions=Index vector (dialog)  Indices=1  OutputSizes=1
  cfblk5 : Bias  Bias=[917769055.319509]
  cfblk6 : Rounding
  cfblk7 : Constant  Value=[-150653421.188522]  SampleTime=1
  cfblk2 : Outport
  cfblk11 : Outport  Port=2
  wires:
  cfblk7/1 -> cfblk4/1
  cfblk3/1 -> cfblk2/1
  cfblk4/1 -> cfblk5/1
  cfblk8/1 -> cfblk4/2
  cfblk10/1 -> cfblk11/1
  cfblk9/1 -> cfblk6/1
  cfblk1/1 -> cfblk3/1
  cfblk6/1 -> cfblk3/2

== system sampleModel153_pp/cfblk60/cfblk8 ==
  cfblk1 : Inport
  cfblk6 : Inport  Port=2
  cfblk7 : Inport  Port=3
  cfblk3 : Bias  Bias=[-106833532.070918]
  cfblk4 : Rounding
  cfblk5 : Product
  cfblk2 : Outport
  wires:
  cfblk7/1 -> cfblk5/1
  cfblk4/1 -> cfblk2/1
  cfblk5/1 -> cfblk3/1
  cfblk6/1 -> cfblk4/1
  cfblk1/1 -> cfblk5/2

== system sampleModel153_pp/cfblk60/cfblk9 ==
  cfblk1 : Inport
  cfblk10 : Inport  Port=2
  cfblk11 : Inport  Port=3
  cfblk3 : simulink/Discrete/Difference  ICPrevInput=0.0  OutMin=[]  OutMax=[]  OutDataTypeStr=Inherit: Inherit via back propagation  OutDataType=fixdt(1, 16)  OutScaling=2^-10  DoSatur=off
  cfblk4 : DiscreteZeroPole  Poles=[0 0.5]  Gain=1
  cfblk5 : Delay  DelayLengthSource=Input port  SampleTime=1
      settings: InputPortMap=u0,p1
  cfblk6 : DiscreteIntegrator  ICPrevOutput=DiscIntNeverNeededParam  ICPrevScaledInput=DiscIntNeverNeededParam
  cfblk7 : Gain  Gain=[58508049.064386]
  cfblk8 : Constant  Value=[-982332398.200745]  SampleTime=1
  cfblk9 : Constant  Value=[864491933.410831]  SampleTime=1
  cfblk2 : Outport
  cfblk12 : Outport  Port=2
  cfblk13 : Outport  Port=3
  wires:
  cfblk8/1 -> cfblk12/1
  cfblk11/1 -> cfblk7/1
  cfblk5/1 -> cfblk2/1
  cfblk4/1 -> cfblk5/1
  cfblk10/1 -> cfblk4/1
  cfblk7/1 -> cfblk5/2
  cfblk1/1 -> cfblk3/1
  cfblk3/1 -> cfblk6/1
  cfblk9/1 -> cfblk13/1

== system sampleModel153_pp/cfblk61/cfblk9 ==
  cfblk1 : Inport
  cfblk10 : Inport  Port=2
  cfblk11 : Inport  Port=3
  cfblk12 : Inport  Port=4
  cfblk13 : Delay  SampleTime=1
  cfblk3 : simulink/Discrete/Tapped Delay  vinit=0.0  samptime=-1  NumDelays=1  DelayOrder=Oldest  includeCurrent=off
  cfblk4 : Delay  SampleTime=1
  cfblk5 : MinMax  Function=max  Inputs=3
  cfblk6 : Polyval  Coefs=[ +2.081618890e-019, -1.441693666e-014, +4.719686976e-010, -8.536869453e-006, +1.621573104e-001, -8.087801117e+001 ]
  cfblk7 : Sqrt  SaturateOnIntegerOverflow=on
  cfblk8 : Product
  cfblk9 : Constant  Value=[-858290224.581137]  SampleTime=1
  cfblk2 : Outport
  wires:
  cfblk11/1 -> cfblk5/1
  cfblk6/1 -> cfblk3/1
  cfblk10/1 -> cfblk6/1
  cfblk3/1 -> cfblk2/1
  cfblk9/1 -> cfblk5/2
  cfblk12/1 -> cfblk7/1
  cfblk7/1 -> cfblk8/1
  cfblk5/1 -> cfblk8/2
  cfblk1/1 -> cfblk4/1
  cfblk8/1 -> cfblk13/1
  cfblk13/1 -> cfblk5/3

== system sampleModel153_pp/cfblk63/cfblk10 ==
  cfblk1 : Inport
  cfblk10 : Bias  Bias=[-495840406.587390]
  cfblk11 : Rounding
  cfblk12 : Constant  Value=[-895157774.105314]  SampleTime=1
  cfblk3 : Delay  ShowEnablePort=on  SampleTime=1
      settings: InputPortMap=u0,e6
  cfblk4 : simulink/Discrete/Transfer Fcn First Order  PoleZ=0.95  ICPrevOutput=0.0  DoSatur=off
  cfblk5 : pid_lib/PID Controller  Controller=PID  Form=Parallel  TimeDomain=Discrete-time  UseExternalTs=off  SampleTime=1  IntegratorMethod=Forward Euler  FilterMethod=Forward Euler  ControllerParametersSource=internal  P=1  I=1  D=0  UseFilter=on  N=100  TunerSelectOption=Transfer Function Based (PID Tuner App)  InitialConditionSource=internal  InitialConditionForIntegrator=0  InitialConditionForFilter=0  DifferentiatorICPrevScaledInput=0  ExternalReset=none  TrackingMode=off  Kt=1  LimitOutput=off  SatLimitsSource=internal  UpperSaturationLimit=inf  LowerSaturationLimit=-inf  LinearizeAsGain=off  AntiWindupMode=none  Kb=1  POutMin=[]  POutMax=[]  IOutMin=[]  IOutMax=[]  DOutMin=[]  DOutMax=[]  NOutMin=[]  NOutMax=[]  SumOutMin=[]  SumOutMax=[]  SaturationOutMin=[]  SaturationOutMax=[]  PParamMin=[]  PParamMax=[]  IParamMin=[]  IParamMax=[]  DParamMin=[]  DParamMax=[]  NParamMin=[]  NParamMax=[]  KbParamMin=[]  KbParamMax=[]  KtParamMin=[]  KtParamMax=[]  KbOutMin=[]  KbOutMax=[]  KtOutMin=[]  KtOutMax=[]  IntegratorOutMin=[]  IntegratorOutMax=[]  FilterOutMin=[]  FilterOutMax=[]  SumI1OutMin=[]  SumI1OutMax=[]  SumI2OutMin=[]  SumI2OutMax=[]  SumI3OutMin=[]  SumI3OutMax=[]  SumI4OutMin=[]  SumI4OutMax=[]  SumDOutMin=[]  SumDOutMax=[]  DifferentiatorOutMin=[]  DifferentiatorOutMax=[]  FilterDiffOutCoefMin=[]  FilterDiffOutCoefMax=[]  ReciprocalOutMin=[]  ReciprocalOutMax=[]  SumDenOutMin=[]  SumDenOutMax=[]  SumNumOutMin=[]  SumNumOutMax=[]  DivideOutMin=[]  DivideOutMax=[]  UdiffTsProdOutMin=[]  UdiffTsProdOutMax=[]  NTsProdOutMin=[]  NTsProdOutMax=[]  UintegralTsProdOutMin=[]  UintegralTsProdOutMax=[]  UngainTsProdOutMin=[]  UngainTsProdOutMax=[]  IntegratorContinuousStateAttributes=''  IntegratorStateMustResolveToSignalObject=off  IntegratorRTWStateStorageClass=Auto  FilterContinuousStateAttributes=''  FilterStateMustResolveToSignalObject=off  FilterRTWStateStorageClass=Auto  ParallelPVariant=InternalParameters  IdealPVariant=Disabled  IVariant=InternalParameters  DVariant=InternalParameters  IntegratorVariant=Discrete  SatVariant=Disabled  AWVariant=Passthrough  PCopyVariant=Disabled  TRVariant=Disabled  FdbkBlocksVariant=Forward  IdealPFdbkVariant=Disabled  SatFdbkVariant=Disabled  DerivativeFilterVariant=ForwardEulerFilter  NVariant=InternalParameters  NCopyVariant=Disabled  FilterICVariant=InternalICsFilter  IntegratorICVariant=InternalICs  ExternalResetVariant=Disabled  TRSumVariant=Passthrough  SumFdbkVariant=Disabled  SumVariant=Sum_PID  TsampFilterVariant=InternalTs  TsampNgainVariant=Passthrough  TsampIntegralVariant=Passthrough  ExternalSaturationOutDataTypeStr=Inherit: Same as second input
  cfblk6 : Sum  Inputs=+
  cfblk7 : Rounding
  cfblk8 : Assignment  DiagnosticForDimensions=Warning  IndexOptions=Index vector (dialog)  Indices=1  OutputSizes=1
  cfblk9 : PermuteDimensions
  cfblk2 : Outport
  cfblk13 : Outport  Port=2
  cfblk14 : Outport  Port=3
  cfblk15 : Outport  Port=4
  wires:
  cfblk7/1 -> cfblk8/1
  cfblk8/1 -> cfblk14/1
  cfblk1/1 -> cfblk5/1
  cfblk4/1 -> cfblk7/1, cfblk11/1, cfblk6/1
  cfblk12/1 -> cfblk4/1
  cfblk6/1 -> cfblk3/1
  cfblk5/1 -> cfblk13/1, cfblk10/1
  cfblk11/1 -> cfblk3/2
  cfblk9/1 -> cfblk8/2
  cfblk10/1 -> cfblk15/1, cfblk9/1
  cfblk3/1 -> cfblk2/1
